simulink model "FSM_mod"  (R2023a)
settings: Solver=FixedStepDiscrete  StartTime=0.0  StopTime=10.0  FixedStep=0.1  RelTol=1e-3  EnableMultiTasking=on
settings Model: Creator=sanbaosu  LastModifiedBy=sanbaosu
settings SolverCC: AlgebraicLoopSolver=TrustRegion  AutoInsertRateTranBlk=on
settings DataIOCC: LimitDataPoints=on
settings OptimizationCC: LifeSpan=inf
settings DebuggingCC: UnconnectedInputMsg=warning  UnconnectedOutputMsg=warning  UnconnectedLineMsg=warning  AllowSymbolicDim=off  SFUnexpectedBacktrackingDiag=warning  SFNoUnconditionalDefaultTransitionDiag=warning  SFExecutionAtInitializationDiag=none  ArithmeticOperatorsInVariantConditions=warning
settings ModelReferenceCC: EnableRefExpFcnMdlSchedulingChecks=on
settings SFSimCC: SimUseLocalCustomCode=off  CustomCodeUndefinedFunction=UseInterfaceOnly
settings RTWCC: RTWUseLocalCustomCode=off  DLArmComputeVersion=19.05
settings CodeAppCC: StateflowObjectComments=on
settings GRTTargetCC: TargetLangStandard=C89/C90 (ANSI)
settings ConfigComp: CovMetricSettings=dw  CovSaveCumulativeToWorkspaceVar=on  CovSaveSingleToWorkspaceVar=on  CovExternalEMLEnable=off  CovSFcnEnable=off

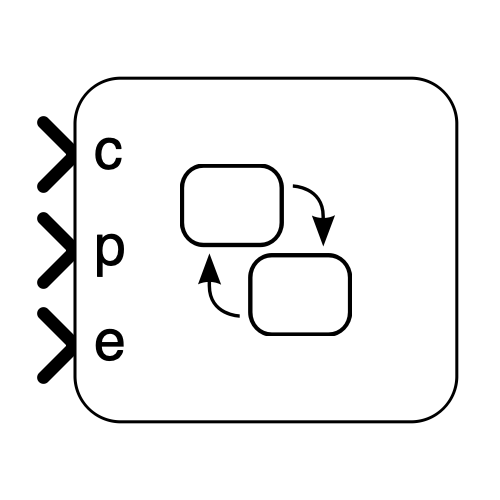
[thumbnail: Simulink's stored preview of the top-level diagram]
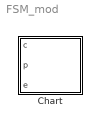
== system FSM_mod ==
  Chart : Stateflow chart  TreatAsAtomicUnit=on

== stateflow chart FSM_mod/Chart ==
  state PL
  state PR
  state L
  state ACC
  state R
  state BL
  state BR
  (junction 55) -> PR [order 2] : [c == -1, p == 0, e == 0]
  (junction 50) -> PL [order 2] : [c == 1, p == 0, e == 0]
  PL -> (junction 41)
  BL -> PL : [c == 1, p == 0]
  BR -> PR : [c == -1, p == 0]
  PR -> (junction 56)
  (junction 19) -> PL [order 2] : [c == 1]
  (junction 19) -> PR [order 1] : [c == -1]
  (junction 56) -> ACC [order 2] : [c ~= -1]
  (junction 56) -> R [order 1] : [c == -1, e == 1]
  (junction 41) -> L [order 1] : [c == 1, e == 1]
  (junction 41) -> ACC [order 2] : [c ~= 1]
  ACC -> (junction 19)
  (default) -> ACC
  L -> (junction 50)
  (junction 50) -> ACC [order 3] : [c == 1, p == 1]
  (junction 55) -> ACC [order 3] : [c == -1, p == 1]
  R -> (junction 55)
  (junction 50) -> BL [order 1] : [c == 1, p == 0.5, e == 0]
  (junction 55) -> BR [order 1] : [c == -1, p == 0.5, e == 0]
  data: c input; p input; e input
